simulink subsystem "Guidance_CMDs"  (R2025b)
settings: Solver=VariableStepAuto  StartTime=0.0  StopTime=10.0  RelTol=1e-3
settings Model: Creator=cdriggs  LastModifiedBy=cdriggs

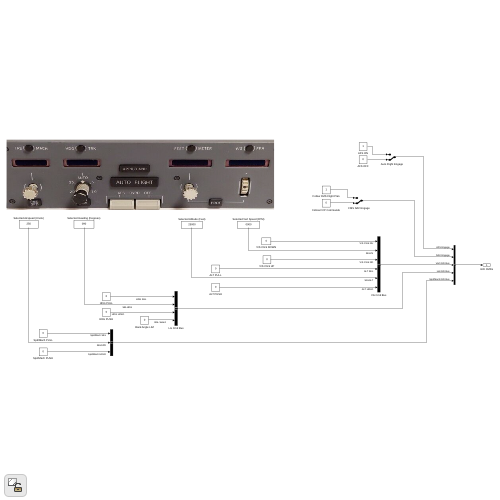
[thumbnail: Simulink's stored preview of the top-level diagram]
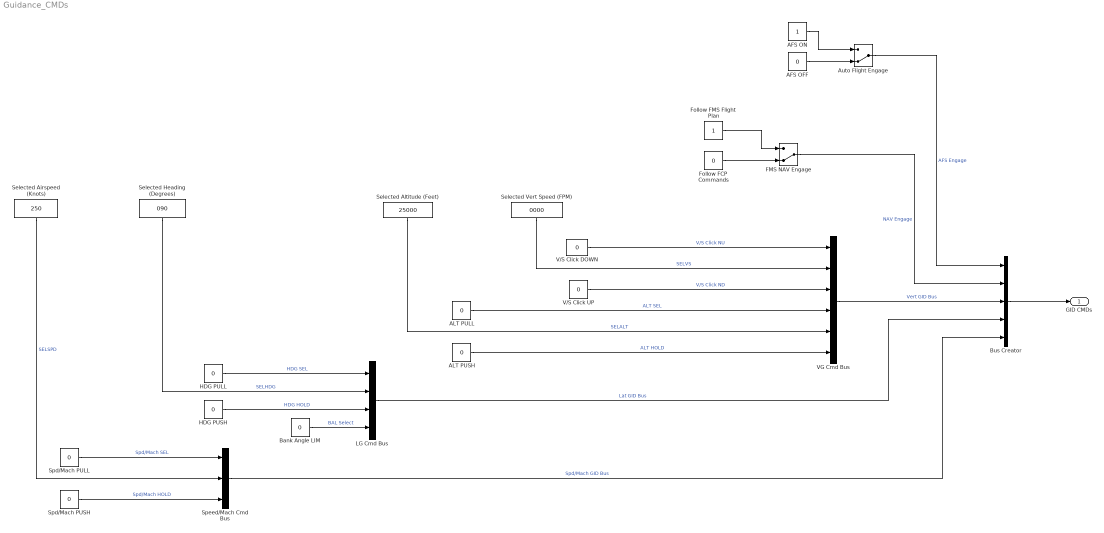
== system Guidance_CMDs ==
  AFS OFF : Constant  Value=0
  AFS ON : Constant
  ALT PULL : Constant  Value=0
  ALT PUSH : Constant  Value=0
  Auto Flight Engage : ManualSwitch  CurrentSetting=0
  Bank Angle LIM : Constant  Value=0
  Bus Creator : BusCreator  Inputs=5
  FMS NAV Engage : ManualSwitch  CurrentSetting=0
  Follow FCP Commands : Constant  Value=0
  Follow FMS Flight Plan : Constant
  HDG PULL : Constant  Value=0
  HDG PUSH : Constant  Value=0
  LG Cmd Bus : BusCreator  Inputs=4
  Selected Airspeed (Knots) : Constant  Value=250
  Selected Altitude (Feet) : Constant  Value=25000
  Selected Heading (Degrees) : Constant  Value=090
  Selected Vert Speed (FPM) : Constant  Value=0000
  Spd/Mach PULL : Constant  Value=0
  Spd/Mach PUSH : Constant  Value=0
  Speed/Mach Cmd Bus : BusCreator  Inputs=3
  V/S Click DOWN : Constant  Value=0
  V/S Click UP : Constant  Value=0
  VG Cmd Bus : BusCreator  Inputs=6
  GID CMDs : Outport
  wires:
  Bus Creator/1 -> GID CMDs/1
  VG Cmd Bus/1 -> Bus Creator/3  "Vert GID Bus"
  LG Cmd Bus/1 -> Bus Creator/4  "Lat GID Bus"
  Speed/Mach Cmd Bus/1 -> Bus Creator/5  "Spd/Mach GID Bus"
  Selected Altitude (Feet)/1 -> VG Cmd Bus/5  "SELALT"
  Selected Vert Speed (FPM)/1 -> VG Cmd Bus/2  "SELVS"
  Selected Heading (Degrees)/1 -> LG Cmd Bus/2  "SELHDG"
  Selected Airspeed (Knots)/1 -> Speed/Mach Cmd Bus/2  "SELSPD"
  Auto Flight Engage/1 -> Bus Creator/1  "AFS Engage"
  AFS ON/1 -> Auto Flight Engage/1
  AFS OFF/1 -> Auto Flight Engage/2
  Follow FMS Flight Plan/1 -> FMS NAV Engage/1
  Follow FCP Commands/1 -> FMS NAV Engage/2
  FMS NAV Engage/1 -> Bus Creator/2  "NAV Engage"
  Bank Angle LIM/1 -> LG Cmd Bus/4  "BAL Select"
  HDG PULL/1 -> LG Cmd Bus/1  "HDG SEL"
  HDG PUSH/1 -> LG Cmd Bus/3  "HDG HOLD"
  Spd/Mach PUSH/1 -> Speed/Mach Cmd Bus/3  "Spd/Mach HOLD"
  Spd/Mach PULL/1 -> Speed/Mach Cmd Bus/1  "Spd/Mach SEL"
  V/S Click DOWN/1 -> VG Cmd Bus/1  "V/S Click NU"
  V/S Click UP/1 -> VG Cmd Bus/3  "V/S Click ND"
  ALT PULL/1 -> VG Cmd Bus/4  "ALT SEL"
  ALT PUSH/1 -> VG Cmd Bus/6  "ALT HOLD"
